simulink model "ABDELSAMEI_MOHAMED_SIMULINK"  (R2018b)
settings: Solver=VariableStepAuto  StartTime=0.0  StopTime=10.0  RelTol=1e-3
values from neighbouring files (symbols this model uses):
  denGs = [1 11 10 0]    [ABDESAMEI_MOHAMED_WORKSPACE.mat]
  denRs = [1 14.58]    [ABDESAMEI_MOHAMED_WORKSPACE.mat]
  denRz = [1 -0.232701212062]    [ABDESAMEI_MOHAMED_WORKSPACE.mat]
  k = 13    [ABDESAMEI_MOHAMED_WORKSPACE.mat]
  numGs = [0 0 0 39.5]    [ABDESAMEI_MOHAMED_WORKSPACE.mat]
  numRs = [1 1.44]    [ABDESAMEI_MOHAMED_WORKSPACE.mat]
  numRz = [1 -0.92421740366]    [ABDESAMEI_MOHAMED_WORKSPACE.mat]
  T = 0.1    [ABDESAMEI_MOHAMED_WORKSPACE.mat]
settings Model: Creator=M  LastModifiedBy=M

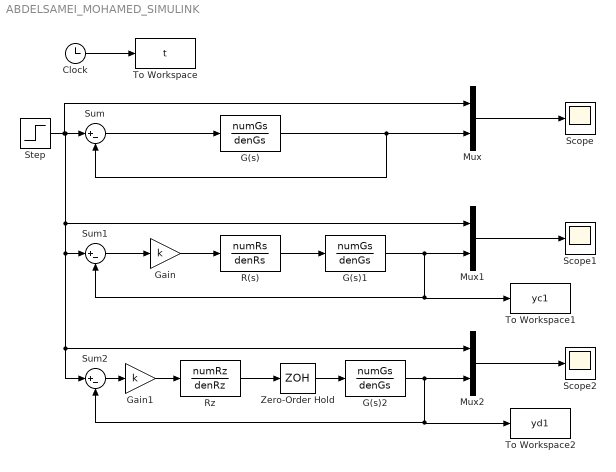
== system ABDELSAMEI_MOHAMED_SIMULINK ==
  Clock : Clock
  G(s) : TransferFcn  Numerator=numGs  Denominator=denGs
  G(s)1 : TransferFcn  Numerator=numGs  Denominator=denGs
  G(s)2 : TransferFcn  Numerator=numGs  Denominator=denGs
  Gain : Gain  Gain=k
  Gain1 : Gain  Gain=k
  Mux : Mux  Inputs=2
  Mux1 : Mux  Inputs=2
  Mux2 : Mux  Inputs=2
  R(s) : TransferFcn  Numerator=numRs  Denominator=denRs
  Rz : DiscreteTransferFcn  Numerator=numRz  Denominator=denRz  SampleTime=T
  Scope : Scope
  Scope1 : Scope
  Scope2 : Scope
  Step : Step  Time=0  SampleTime=0
  Sum : Sum  Inputs=|+-
  Sum1 : Sum  Inputs=|+-
  Sum2 : Sum  Inputs=|+-
  To Workspace : ToWorkspace  VariableName=t  SampleTime=-1
  To Workspace1 : ToWorkspace  VariableName=yc1  SampleTime=-1
  To Workspace2 : ToWorkspace  VariableName=yd1  SampleTime=-1
  Zero-Order Hold : ZeroOrderHold  SampleTime=T
  wires:
  Sum/1 -> G(s)/1
  G(s)/1 -> Sum/2, Mux/2
  Mux/1 -> Scope/1
  Clock/1 -> To Workspace/1
  Mux1/1 -> Scope1/1
  G(s)1/1 -> Mux1/2, Sum1/2, To Workspace1/1
  R(s)/1 -> G(s)1/1
  Gain/1 -> R(s)/1
  Sum1/1 -> Gain/1
  Sum2/1 -> Gain1/1
  Gain1/1 -> Rz/1
  Rz/1 -> Zero-Order Hold/1
  Step/1 -> Mux/1, Mux1/1, Mux2/1, Sum2/1, Sum1/1, Sum/1
  G(s)2/1 -> To Workspace2/1, Sum2/2, Mux2/2
  Mux2/1 -> Scope2/1
  Zero-Order Hold/1 -> G(s)2/1
